simulink model "VehicleDynamicsRing"  (R2020a)
settings: Solver=FixedStepDiscrete  StartTime=0.0  StopTime=10.0  FixedStep=ModelSimTime  RelTol=1e-3  EnableMultiTasking=on
PostLoadFcn:
  | , if any(exist('dsrtsu_mdlpostloadfcn', 'file') ~= 0), dsrtsu_mdlpostloadfcn('Execute', bdroot); end,
InitFcn:
  | , if any(exist('rtifpga_mdlclblib', 'file') ~= 0), rtifpga_mdlclblib('Init', bdroot); end,
undefined symbols (not defined in the file): DRIVE_MODE, VDR
libraries: simulink x4
(part 1 of 2)
settings Model: DSRTSU_INTERNAL_RTI_VER=560  DSRTSU_INTERNAL_RTI_TYPE=rti1401  RTICANMMDATA=struct('GeneralSetupData',struct('modelroot','C:\Users\harjo\Git\MACFormulaGit\MicroAutobox\rings\Vehicle_Dynamics_Ring','generalsettings',struct('filesettings',struct('destfolder',struct('Name','RTICANMM_FILES','Check',1),'buildfolder',struct('Name','.','Check',1),'AbsDestfolder',struct('Name','C:\Users\harjo\Git\MACFormulaGit\MicroAutobox\rings\Vehicle_Dynamics_Ring\RTICANMM_FILES'),'AbsBuildfolder',struct('Name','C:\Users\harjo\Git\MACFormulaGit\MicroAutobox\rings\Vehicle_Dynamics_Ring'))),'options',struct('addpaths',1,'rmpaths',1,'addtrcexclusion',true,'cannavigator',struct('checkmonitoring',0),'show_usrtrc',0,'use_usrtrc',0),'advanced',struct('options',ones(1,100)),'MPSetup',{{}},'RTI',struct('Type','RTI1401','Ver','7.14','Date','02-May-2020'),'modelname','VehicleDynamicsRing','block','VehicleDynamicsRing'))  DSRTSU_INTERNAL_RTIFPGA=160  Creator=Harjot  LastModifiedBy=Harjot
settings DebuggingCC: AlgebraicLoopMsg=error  ArtificialAlgebraicLoopMsg=error  MinStepSizeMsg=error  SFUnexpectedBacktrackingDiag=warning  SFNoUnconditionalDefaultTransitionDiag=warning  SFExecutionAtInitializationDiag=none  ArithmeticOperatorsInVariantConditions=warning
settings HardwareCC: ProdBitPerPointer=32  ProdBitPerSizeT=32  ProdBitPerPtrDiffT=32  ProdLargestAtomicInteger=Integer  ProdEndianess=BigEndian  ProdWordSize=32  ProdHWDeviceType=Custom Processor->Custom  TargetIntDivRoundTo=Zero  TargetEndianess=BigEndian  TargetHWDeviceType=Custom Processor->Custom
settings SFSimCC: SimUseLocalCustomCode=off  MATLABDynamicMemAlloc=off  CustomCodeUndefinedFunction=UseInterfaceOnly
settings RTWCC: Description=dSPACE DS1401 Hardware Platform  SystemTargetFile=rti1401.tlc  MakeCommand=make_rti  TemplateMakefile=rti1401.tmf  RTWUseLocalCustomCode=off
settings CodeAppCC: StateflowObjectComments=on
settings STFCustomTargetCC: UtilityFuncGeneration=Shared location  ParMdlRefBuildCompliant=on  SystemTargetFile=rti1401.tlc
settings GRTTargetCC: TargetLangStandard=C89/C90 (ANSI)  UtilityFuncGeneration=Shared location  CompOptLevelCompliant=off  ConcurrentExecutionCompliant=off  CombineOutputUpdateFcns=off  MatFileLogging=off  CPPClassGenCompliant=off  UseToolchainInfoCompliant=off
settings ConfigComp: CovMetricSettings=dw  CovHtmlReporting=on  CovSaveCumulativeToWorkspaceVar=on  CovSaveSingleToWorkspaceVar=on  CovExternalEMLEnable=off

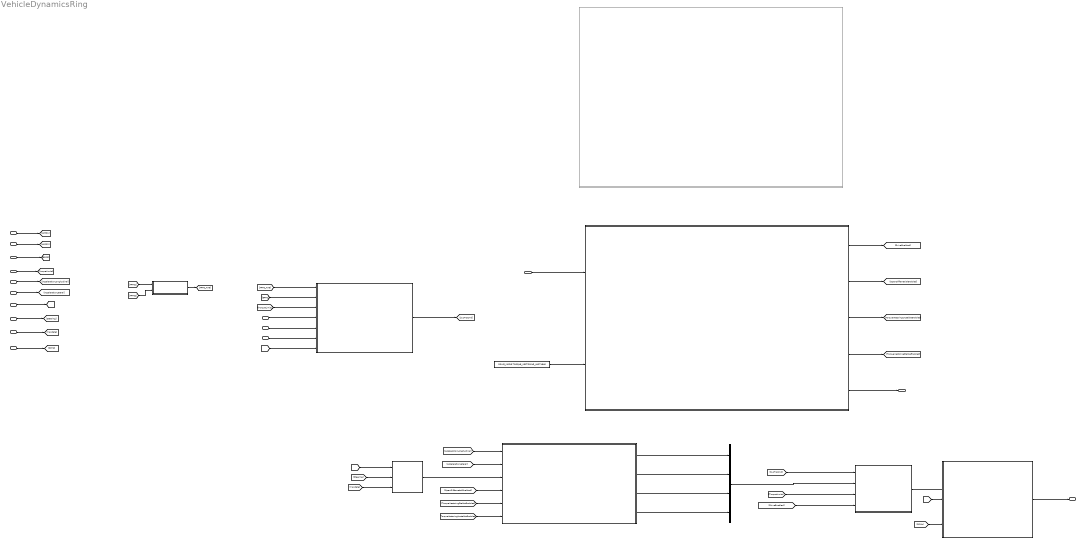
== system VehicleDynamicsRing ==
  VdrModeRequest : Inport  OutDataTypeStr=Enum: MSR_REQUEST
  APPS1 [%]1 : Inport  Port=2  OutDataTypeStr=double
  APPS2 [%]1 : Inport  Port=3  OutDataTypeStr=double
  BPPS : Inport  Port=4  OutDataTypeStr=double
  TorqueLimits : Inport  Port=5  OutDataTypeStr=Bus: TorqueLimits
  AccelerationLongitudinal : Inport  Port=6  OutDataTypeStr=double
  AccelerationLateral : Inport  Port=7  OutDataTypeStr=double
  VehicleSpeed : Inport  Port=8
  SteeringAngle : Inport  Port=9
  YawRate : Inport  Port=10
  ChargeCurrentLimit : Inport  Port=11  OutDataTypeStr=double
  DischargeCurrentLimit : Inport  Port=12  OutDataTypeStr=double
  AccumulatorVoltage : Inport  Port=13
  MotorRPMs : Inport  Port=14  OutDataTypeStr=Bus: MotorRPMs
  APPS Average : Subsystem
  Bus Creator1 : BusCreator  Inputs=4
  Constant1 : Constant  Value=DRIVE_MODE.TORQUE_VECTORING_UNSTABLE
  PedalMapping : ModelReference  ModelNameDialog=PedalMapping.slx  SimulationMode=Normal  ModelReferenceVersion=1.20
  TorqueVectoring : Subsystem
  Traction Control : Subsystem
  VDR Mode Selection : Stateflow chart  TreatAsAtomicUnit=on
  VDR Mode Selection1 : Stateflow chart  Commented=on  TreatAsAtomicUnit=on
  Yaw error subsystem : Subsystem
  torque_distribution_mapping : MATLAB Function  TreatAsAtomicUnit=on
  VdrStatus : Outport  OutDataTypeStr=Enum: RING_STATUS  VectorParamsAs1DForOutWhenUnconnected=off
  TorqueRequests : Outport  Port=2  OutDataTypeStr=Bus: TorqueRequests  VectorParamsAs1DForOutWhenUnconnected=off
  wires:
  VdrModeRequest/1 -> VDR Mode Selection/1(VdrModeRequest)
  AccelerationLongitudinal/1 -> [AccelerationLongitudinal]
  APPS1 [%]1/1 -> [APPS1]
  VehicleSpeed/1 -> [Speed]
  Constant1/1 -> VDR Mode Selection/2(DrivingMode)
  PedalMapping/1 -> [SysTrqCmd]
  APPS Average/1(APPS) -> [APPS_AVG]
  [APPS2] -> APPS Average/2(APPS2)
  APPS2 [%]1/1 -> [APPS2]
  [APPS1] -> APPS Average/1(APPS1)
  BPPS/1 -> [BPPS]
  AccelerationLateral/1 -> [AccelerationLateral]
  DischargeCurrentLimit/1 -> PedalMapping/5
  [APPS_AVG] -> PedalMapping/1
  [BPPS] -> PedalMapping/2
  AccumulatorVoltage/1 -> PedalMapping/6
  [Speed] -> PedalMapping/7
  [TorqueLimits] -> PedalMapping/3
  ChargeCurrentLimit/1 -> PedalMapping/4
  [SysTrqCmd] -> torque_distribution_mapping/1(systemTorque)
  TorqueLimits/1 -> [TorqueLimits]
  [TorqueLimits] -> torque_distribution_mapping/3(torqueLimits)
  Bus Creator1/1 -> torque_distribution_mapping/2(torqueFactors)
  VDR Mode Selection/5(VdrStatus) -> VdrStatus/1  "VDR_Status"
  VDR Mode Selection/4(TorqueVectoringStableEnabled) -> [TorqueVectoringStableEnabled]
  VDR Mode Selection/2(OpenDifferentialEnabled) -> [OpenDiffernetialEnabled]
  [TorqueVectoringStableEnabled] -> TorqueVectoring/5(TorqueVectoringStableEnabled)
  VDR Mode Selection/3(TorqueVectoringUnstableEnabled) -> [TorqueVectoringUnstableEnabled]
  [TorqueVectoringUnstableEnabled] -> TorqueVectoring/6(TorqueVectoringUnstableEnabled)
  Yaw error subsystem/1(Yaw error) -> TorqueVectoring/3(YawError)
  [AccelerationLongitudinal] -> TorqueVectoring/1("AccelerationLongitudinal ")
  [AccelerationLateral] -> TorqueVectoring/2(AccelerationLateral)
  VDR Mode Selection/1(DriveEnabled) -> [DriveEnabled]
  [OpenDiffernetialEnabled] -> TorqueVectoring/4(TorqueVectoringStableEnabled1)
  [Speed] -> Yaw error subsystem/1(Car_speed)
  SteeringAngle/1 -> [Steering]
  [Steering] -> Yaw error subsystem/2(Steering_angle)
  [YawRate] -> Yaw error subsystem/3("Estimated yaw rate ")
  YawRate/1 -> [YawRate]
  [DriveEnabled] -> torque_distribution_mapping/4(driveEnabled)
  TorqueVectoring/1(TorqueScaleRearLeft) -> Bus Creator1/1
  TorqueVectoring/2(TorqueScaleRearRight) -> Bus Creator1/2
  TorqueVectoring/3(TorqueScaleFrontLeft) -> Bus Creator1/3
  TorqueVectoring/4(TorqueScaleFrontRight) -> Bus Creator1/4
  [Speed] -> Traction Control/2(Speed)
  [RPMs] -> Traction Control/3(In3)
  MotorRPMs/1 -> [RPMs]
  Traction Control/1(FinalTorqueRequest) -> TorqueRequests/1
  torque_distribution_mapping/1(torqueRequests) -> Traction Control/1(PreTractionControlTorqueRequest)

== system VehicleDynamicsRing/APPS Average ==
  APPS1 : Inport
  APPS2 : Inport  Port=2
  Add : Sum
  Constant : Constant  Value=2
  Divide : Product  Inputs=*/
  APPS : Outport  VectorParamsAs1DForOutWhenUnconnected=off
  wires:
  Divide/1 -> APPS/1
  APPS2/1 -> Add/2
  APPS1/1 -> Add/1
  Add/1 -> Divide/1
  Constant/1 -> Divide/2

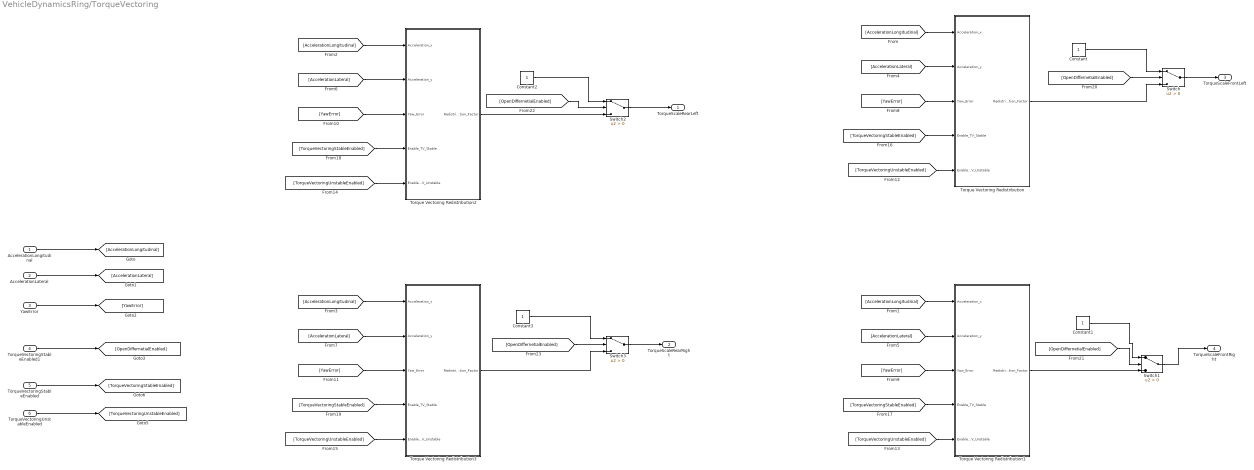
== system VehicleDynamicsRing/TorqueVectoring ==
  "AccelerationLongitudinal " : Inport
  AccelerationLateral : Inport  Port=2
  YawError : Inport  Port=3
  TorqueVectoringStableEnabled1 : Inport  Port=4
  TorqueVectoringStableEnabled : Inport  Port=5
  TorqueVectoringUnstableEnabled : Inport  Port=6
  Constant{,1..3} (4 alike) : Constant
  Switch{,1..3} (4 alike) : Switch  Criteria=u2 > Threshold
  Torque Vectoring Redistribution : Subsystem  AncestorBlock=TorqueVectoringAlgorithmLib/Torque Vectoring Redistribution  mask{wheel_1=Front, wheel_2=Left}
      mask prompts: wheel_1 "Front or Rear Wheel"; wheel_2 "Left or Right Wheel"
      mask init:
      | %Front vs Rear Modifier
      | if(wheel_1 == 1) %Front Wheel
      |     stable_longitudinal_mod = -1;
      | else %Rear Wheel
      |     stable_longitudinal_mod = 1;
      | end
      | 
      | %Left vs Rear Modifier
      | if(wheel_2 == 1) %Left Wheel
      |     unstable_mod = -1;
      |     stable_lateral_mod = -1;
      | else %Right Wheel
      |     unstable_mod = 1;
      |     stable_lateral_mod = 1;
      | end
      mask TypeOptions wheel_1: Front | Rear
      mask TypeOptions wheel_2: Left | Right
      mask DialogControl DescGroupVar Prompt: Torque Vectoring Configurations
      mask DialogControl DescTextVar Prompt: Select the wheel for the torque vectoring configuration.
  Torque Vectoring Redistribution1 : Subsystem  AncestorBlock=TorqueVectoringAlgorithmLib/Torque Vectoring Redistribution  mask{wheel_1=Front, wheel_2=Right}
      mask prompts: wheel_1 "Front or Rear Wheel"; wheel_2 "Left or Right Wheel"
      mask init: same as VehicleDynamicsRing/TorqueVectoring/Torque Vectoring Redistribution
      mask TypeOptions wheel_1: Front | Rear
      mask TypeOptions wheel_2: Left | Right
      mask DialogControl DescGroupVar Prompt: Torque Vectoring Configurations
      mask DialogControl DescTextVar Prompt: Select the wheel for the torque vectoring configuration.
  Torque Vectoring Redistribution2 : Subsystem  AncestorBlock=TorqueVectoringAlgorithmLib/Torque Vectoring Redistribution  mask{wheel_1=Rear, wheel_2=Left}
      mask prompts: wheel_1 "Front or Rear Wheel"; wheel_2 "Left or Right Wheel"
      mask init: same as VehicleDynamicsRing/TorqueVectoring/Torque Vectoring Redistribution
      mask TypeOptions wheel_1: Front | Rear
      mask TypeOptions wheel_2: Left | Right
      mask DialogControl DescGroupVar Prompt: Torque Vectoring Configurations
      mask DialogControl DescTextVar Prompt: Select the wheel for the torque vectoring configuration.
  Torque Vectoring Redistribution3 : Subsystem  AncestorBlock=TorqueVectoringAlgorithmLib/Torque Vectoring Redistribution  mask{wheel_1=Rear, wheel_2=Right}
      mask prompts: wheel_1 "Front or Rear Wheel"; wheel_2 "Left or Right Wheel"
      mask init: same as VehicleDynamicsRing/TorqueVectoring/Torque Vectoring Redistribution
      mask TypeOptions wheel_1: Front | Rear
      mask TypeOptions wheel_2: Left | Right
      mask DialogControl DescGroupVar Prompt: Torque Vectoring Configurations
      mask DialogControl DescTextVar Prompt: Select the wheel for the torque vectoring configuration.
  TorqueScaleRearLeft : Outport  VectorParamsAs1DForOutWhenUnconnected=off
  TorqueScaleRearRight : Outport  Port=2  VectorParamsAs1DForOutWhenUnconnected=off
  TorqueScaleFrontLeft : Outport  Port=3  VectorParamsAs1DForOutWhenUnconnected=off
  TorqueScaleFrontRight : Outport  Port=4  VectorParamsAs1DForOutWhenUnconnected=off
  wires:
  "AccelerationLongitudinal "/1 -> [AccelerationLongitudinal]
  AccelerationLateral/1 -> [AccelerationLateral]
  YawError/1 -> [YawError]
  TorqueVectoringUnstableEnabled/1 -> [TorqueVectoringUnstableEnabled]
  [AccelerationLongitudinal] -> Torque Vectoring Redistribution2/1(Acceleration_x)
  [AccelerationLongitudinal] -> Torque Vectoring Redistribution3/1(Acceleration_x)
  [AccelerationLateral] -> Torque Vectoring Redistribution2/2(Acceleration_y)
  [AccelerationLateral] -> Torque Vectoring Redistribution3/2(Acceleration_y)
  [YawError] -> Torque Vectoring Redistribution2/3(Yaw_Error)
  [YawError] -> Torque Vectoring Redistribution3/3(Yaw_Error)
  TorqueVectoringStableEnabled/1 -> [TorqueVectoringStableEnabled]
  [TorqueVectoringUnstableEnabled] -> Torque Vectoring Redistribution2/5(Enable_TV_Unstable)
  [TorqueVectoringUnstableEnabled] -> Torque Vectoring Redistribution3/5(Enable_TV_Unstable)
  [TorqueVectoringStableEnabled] -> Torque Vectoring Redistribution2/4(Enable_TV_Stable)
  [TorqueVectoringStableEnabled] -> Torque Vectoring Redistribution3/4(Enable_TV_Stable)
  TorqueVectoringStableEnabled1/1 -> [OpenDiffernetialEnabled]
  [TorqueVectoringStableEnabled] -> Torque Vectoring Redistribution/4(Enable_TV_Stable)
  [TorqueVectoringUnstableEnabled] -> Torque Vectoring Redistribution/5(Enable_TV_Unstable)
  [YawError] -> Torque Vectoring Redistribution/3(Yaw_Error)
  [AccelerationLateral] -> Torque Vectoring Redistribution/2(Acceleration_y)
  [AccelerationLongitudinal] -> Torque Vectoring Redistribution/1(Acceleration_x)
  [TorqueVectoringStableEnabled] -> Torque Vectoring Redistribution1/4(Enable_TV_Stable)
  [YawError] -> Torque Vectoring Redistribution1/3(Yaw_Error)
  [AccelerationLongitudinal] -> Torque Vectoring Redistribution1/1(Acceleration_x)
  [TorqueVectoringUnstableEnabled] -> Torque Vectoring Redistribution1/5(Enable_TV_Unstable)
  [AccelerationLateral] -> Torque Vectoring Redistribution1/2(Acceleration_y)
  [OpenDiffernetialEnabled] -> Switch/2
  Switch/1 -> TorqueScaleFrontLeft/1
  [OpenDiffernetialEnabled] -> Switch1/2
  Switch1/1 -> TorqueScaleFrontRight/1
  Constant1/1 -> Switch1/1
  Torque Vectoring Redistribution1/1(Redistribution_Factor) -> Switch1/3
  Torque Vectoring Redistribution/1(Redistribution_Factor) -> Switch/3
  Constant/1 -> Switch/1
  Constant2/1 -> Switch2/1
  [OpenDiffernetialEnabled] -> Switch2/2
  Switch2/1 -> TorqueScaleRearLeft/1
  Torque Vectoring Redistribution2/1(Redistribution_Factor) -> Switch2/3
  Constant3/1 -> Switch3/1
  [OpenDiffernetialEnabled] -> Switch3/2
  Switch3/1 -> TorqueScaleRearRight/1
  Torque Vectoring Redistribution3/1(Redistribution_Factor) -> Switch3/3

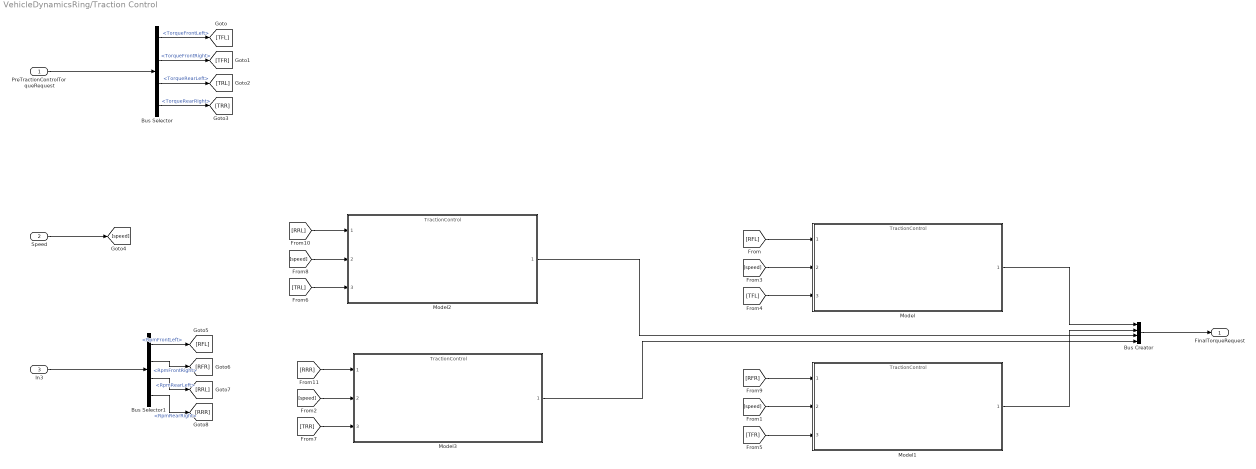
== system VehicleDynamicsRing/Traction Control ==
  PreTractionControlTorqueRequest : Inport
  Speed : Inport  Port=2
  In3 : Inport  Port=3
  Bus Creator : BusCreator  Inputs=4  OutDataTypeStr=Bus: TorqueRequests
  Bus Selector : BusSelector  OutputSignals=TorqueFrontLeft,TorqueFrontRight,TorqueRearLeft,TorqueRearRight
  Bus Selector1 : BusSelector  OutputSignals=RpmFrontLeft,RpmFrontRight,RpmRearLeft,RpmRearRight
  Model{,1..3} (4 alike) : ModelReference  ModelNameDialog=TractionControl.slx  SimulationMode=Normal  ModelReferenceVersion=1.6
  FinalTorqueRequest : Outport  VectorParamsAs1DForOutWhenUnconnected=off
  wires:
  Model3/1 -> Bus Creator/4
  Model2/1 -> Bus Creator/3
  Model1/1 -> Bus Creator/2
  Model/1 -> Bus Creator/1
  Bus Creator/1 -> FinalTorqueRequest/1
  [RFR] -> Model1/1
  [RFL] -> Model/1
  [RRL] -> Model2/1
  [RRR] -> Model3/1
  Bus Selector1/4 -> [RRR]  "<RpmRearRight>"
  Bus Selector1/3 -> [RRL]  "<RpmRearLeft>"
  Bus Selector1/2 -> [RFR]  "<RpmFrontRight>"
  Bus Selector1/1 -> [RFL]  "<RpmFrontLeft>"
  [speed] -> Model1/2
  [speed] -> Model3/2
  [speed] -> Model/2
  [speed] -> Model2/2
  [TRR] -> Model3/3
  [TRL] -> Model2/3
  [TFR] -> Model1/3
  [TFL] -> Model/3
  In3/1 -> Bus Selector1/1
  Speed/1 -> [speed]
  Bus Selector/4 -> [TRR]  "<TorqueRearRight>"
  Bus Selector/3 -> [TRL]  "<TorqueRearLeft>"
  Bus Selector/2 -> [TFR]  "<TorqueFrontRight>"
  Bus Selector/1 -> [TFL]  "<TorqueFrontLeft>"
  PreTractionControlTorqueRequest/1 -> Bus Selector/1

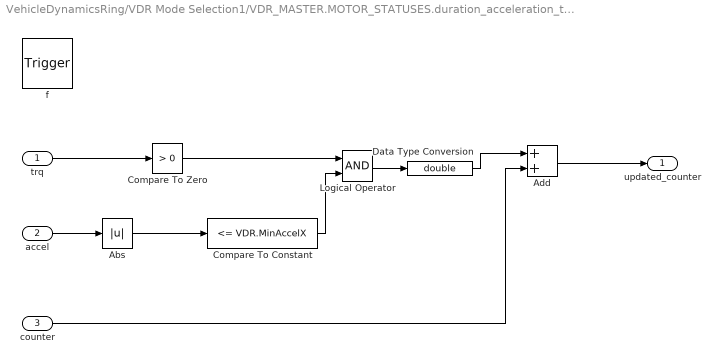
== system VehicleDynamicsRing/VDR Mode Selection1/VDR_MASTER.MOTOR_STATUSES.duration_acceleration_torque_check ==
  trq : Inport  OutDataTypeStr=double  PortDimensions=1
  accel : Inport  Port=2  OutDataTypeStr=double  PortDimensions=1
  counter : Inport  Port=3  OutDataTypeStr=double  PortDimensions=1
  f : TriggerPort  TriggerType=function-call  VariantControl=Variant
      settings: CopyFcn=Stateflow.SLINSF.SimulinkMan.removeBlockPreDeleteFcn  PreDeleteFcn=Stateflow.SLINSF.SimulinkMan.unsafePredeleteFcn
  Abs : Abs
  Add : Sum
  Compare To Constant : simulink/Logic and Bit Operations/Compare To Constant  relop=<=  const=VDR.MinAccelX  OutDataTypeStr=boolean
  Compare To Zero : simulink/Logic and Bit Operations/Compare To Zero  relop=>  OutDataTypeStr=boolean
  Data Type Conversion : DataTypeConversion  OutDataTypeStr=double
  Logical Operator : Logic  AllPortsSameDT=off  OutDataTypeStr=boolean
  updated_counter : Outport  VectorParamsAs1DForOutWhenUnconnected=off
  wires:
  Data Type Conversion/1 -> Add/1
  trq/1 -> Compare To Zero/1
  accel/1 -> Abs/1
  Compare To Zero/1 -> Logical Operator/1
  Compare To Constant/1 -> Logical Operator/2
  Logical Operator/1 -> Data Type Conversion/1
  counter/1 -> Add/2
  Add/1 -> updated_counter/1
  Abs/1 -> Compare To Constant/1

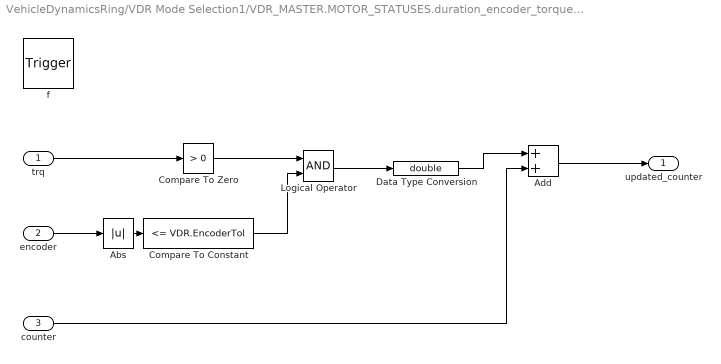
== system VehicleDynamicsRing/VDR Mode Selection1/VDR_MASTER.MOTOR_STATUSES.duration_encoder_torque_check ==
  trq : Inport  OutDataTypeStr=double  PortDimensions=1
  encoder : Inport  Port=2  OutDataTypeStr=double  PortDimensions=1
  counter : Inport  Port=3  OutDataTypeStr=double  PortDimensions=1
  f : TriggerPort  TriggerType=function-call  VariantControl=Variant
      settings: CopyFcn=Stateflow.SLINSF.SimulinkMan.removeBlockPreDeleteFcn  PreDeleteFcn=Stateflow.SLINSF.SimulinkMan.unsafePredeleteFcn
  Abs : Abs
  Add : Sum
  Compare To Constant : simulink/Logic and Bit Operations/Compare To Constant  relop=<=  const=VDR.EncoderTol  OutDataTypeStr=boolean
  Compare To Zero : simulink/Logic and Bit Operations/Compare To Zero  relop=>  OutDataTypeStr=boolean
  Data Type Conversion : DataTypeConversion  OutDataTypeStr=double
  Logical Operator : Logic  AllPortsSameDT=off  OutDataTypeStr=boolean
  updated_counter : Outport  VectorParamsAs1DForOutWhenUnconnected=off
  wires:
  Data Type Conversion/1 -> Add/1
  trq/1 -> Compare To Zero/1
  encoder/1 -> Abs/1
  Compare To Zero/1 -> Logical Operator/1
  Compare To Constant/1 -> Logical Operator/2
  Logical Operator/1 -> Data Type Conversion/1
  counter/1 -> Add/2
  Add/1 -> updated_counter/1
  Abs/1 -> Compare To Constant/1

== system VehicleDynamicsRing/Yaw error subsystem ==
  Car_speed : Inport
  Steering_angle : Inport  Port=2
  "Estimated yaw rate " : Inport  Port=3
  Desired yaw rate calculation : Subsystem
  Subtract : Sum  Inputs=+-
  Yaw rate estimatior : Subsystem  Commented=on
  Yaw error : Outport  VectorParamsAs1DForOutWhenUnconnected=off
  wires:
  Steering_angle/1 -> Desired yaw rate calculation/2(Steering angle)
  Subtract/1 -> Yaw error/1
  "Estimated yaw rate "/1 -> Subtract/2
  Car_speed/1 -> Desired yaw rate calculation/1(Car speed)
  Desired yaw rate calculation/1(Desired yaw rate) -> Subtract/1

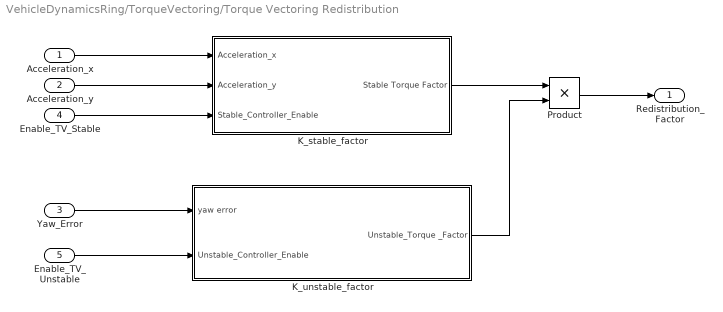
== system VehicleDynamicsRing/TorqueVectoring/Torque Vectoring Redistribution ==
  Acceleration_x : Inport
  Acceleration_y : Inport  Port=2
  Yaw_Error : Inport  Port=3
  Enable_TV_Stable : Inport  Port=4
  Enable_TV_Unstable : Inport  Port=5
  K_stable_factor : Subsystem
  K_unstable_factor : Subsystem
  Product : Product
  Redistribution_Factor : Outport  VectorParamsAs1DForOutWhenUnconnected=off
  wires:
  Enable_TV_Unstable/1 -> K_unstable_factor/2(Unstable_Controller_Enable)
  Enable_TV_Stable/1 -> K_stable_factor/3(Stable_Controller_Enable)
  Product/1 -> Redistribution_Factor/1
  Acceleration_y/1 -> K_stable_factor/2(Acceleration_y)
  Yaw_Error/1 -> K_unstable_factor/1(yaw error)
  Acceleration_x/1 -> K_stable_factor/1(Acceleration_x)
  K_stable_factor/1(Stable Torque Factor) -> Product/1
  K_unstable_factor/1(Unstable_Torque _Factor) -> Product/2

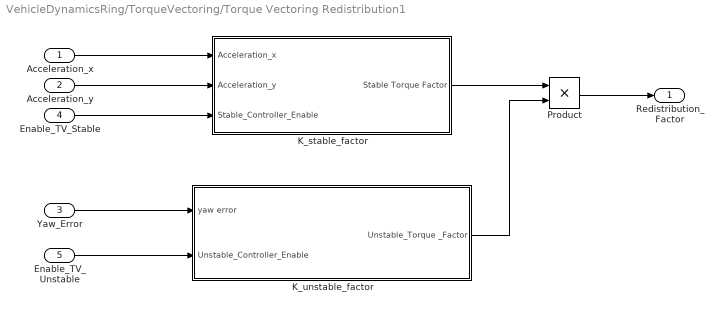
== system VehicleDynamicsRing/TorqueVectoring/Torque Vectoring Redistribution1 ==
  Acceleration_x : Inport
  Acceleration_y : Inport  Port=2
  Yaw_Error : Inport  Port=3
  Enable_TV_Stable : Inport  Port=4
  Enable_TV_Unstable : Inport  Port=5
  K_stable_factor : Subsystem
  K_unstable_factor : Subsystem
  Product : Product
  Redistribution_Factor : Outport  VectorParamsAs1DForOutWhenUnconnected=off
  wires:
  Enable_TV_Unstable/1 -> K_unstable_factor/2(Unstable_Controller_Enable)
  Enable_TV_Stable/1 -> K_stable_factor/3(Stable_Controller_Enable)
  Product/1 -> Redistribution_Factor/1
  Acceleration_y/1 -> K_stable_factor/2(Acceleration_y)
  Yaw_Error/1 -> K_unstable_factor/1(yaw error)
  Acceleration_x/1 -> K_stable_factor/1(Acceleration_x)
  K_stable_factor/1(Stable Torque Factor) -> Product/1
  K_unstable_factor/1(Unstable_Torque _Factor) -> Product/2

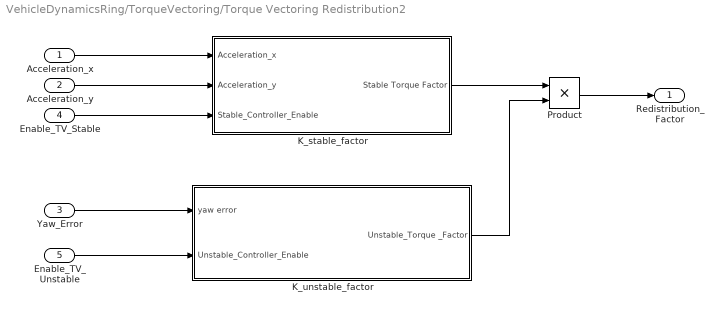
== system VehicleDynamicsRing/TorqueVectoring/Torque Vectoring Redistribution2 ==
  Acceleration_x : Inport
  Acceleration_y : Inport  Port=2
  Yaw_Error : Inport  Port=3
  Enable_TV_Stable : Inport  Port=4
  Enable_TV_Unstable : Inport  Port=5
  K_stable_factor : Subsystem
  K_unstable_factor : Subsystem
  Product : Product
  Redistribution_Factor : Outport  VectorParamsAs1DForOutWhenUnconnected=off
  wires:
  Enable_TV_Unstable/1 -> K_unstable_factor/2(Unstable_Controller_Enable)
  Enable_TV_Stable/1 -> K_stable_factor/3(Stable_Controller_Enable)
  Product/1 -> Redistribution_Factor/1
  Acceleration_y/1 -> K_stable_factor/2(Acceleration_y)
  Yaw_Error/1 -> K_unstable_factor/1(yaw error)
  Acceleration_x/1 -> K_stable_factor/1(Acceleration_x)
  K_stable_factor/1(Stable Torque Factor) -> Product/1
  K_unstable_factor/1(Unstable_Torque _Factor) -> Product/2

== system VehicleDynamicsRing/TorqueVectoring/Torque Vectoring Redistribution3 ==
  Acceleration_x : Inport
  Acceleration_y : Inport  Port=2
  Yaw_Error : Inport  Port=3
  Enable_TV_Stable : Inport  Port=4
  Enable_TV_Unstable : Inport  Port=5
  K_stable_factor : Subsystem
  K_unstable_factor : Subsystem
  Product : Product
  Redistribution_Factor : Outport  VectorParamsAs1DForOutWhenUnconnected=off
  wires:
  Enable_TV_Unstable/1 -> K_unstable_factor/2(Unstable_Controller_Enable)
  Enable_TV_Stable/1 -> K_stable_factor/3(Stable_Controller_Enable)
  Product/1 -> Redistribution_Factor/1
  Acceleration_y/1 -> K_stable_factor/2(Acceleration_y)
  Yaw_Error/1 -> K_unstable_factor/1(yaw error)
  Acceleration_x/1 -> K_stable_factor/1(Acceleration_x)
  K_stable_factor/1(Stable Torque Factor) -> Product/1
  K_unstable_factor/1(Unstable_Torque _Factor) -> Product/2

== system VehicleDynamicsRing/Yaw error subsystem/Desired yaw rate calculation ==
  Car speed : Inport
  Steering angle : Inport  Port=2
  Add : Sum
  "CM to front axel " : Constant  Value=VDR.l_f
  CM to rear axel : Constant  Value=VDR.l_r
  Divide : Product  Inputs=*/
  Product : Product
  Desired yaw rate : Outport  VectorParamsAs1DForOutWhenUnconnected=off
  wires:
  Steering angle/1 -> Product/2
  Add/1 -> Divide/2
  Divide/1 -> Desired yaw rate/1
  Car speed/1 -> Product/1
  Product/1 -> Divide/1
  CM to rear axel/1 -> Add/2
  "CM to front axel "/1 -> Add/1

== system VehicleDynamicsRing/Yaw error subsystem/Yaw rate estimatior ==
  velocity-x : Inport
  steering angle : Inport  Port=2
  Divide : Product  Inputs=*/
  Product : Product
  Trigonometric Function : Trigonometry  Operator=tan
  Wheelbase : Constant  Value=VDR.l
  yaw rate estimate : Outport  VectorParamsAs1DForOutWhenUnconnected=off
  wires:
  steering angle/1 -> Trigonometric Function/1
  velocity-x/1 -> Product/1
  Trigonometric Function/1 -> Product/2
  Product/1 -> Divide/1
  Wheelbase/1 -> Divide/2
  Divide/1 -> yaw rate estimate/1

== system VehicleDynamicsRing/TorqueVectoring/Torque Vectoring Redistribution/K_stable_factor ==
  Acceleration_x : Inport
  Acceleration_y : Inport  Port=2
  Stable_Controller_Enable : Inport  Port=3
  Constant : Constant
  Divide : Product  Inputs=*/
  Switch : Switch  Criteria=u2 > Threshold
  Vehicle Mass : Constant  Value=0.25*VDR.M*VDR.g
  Wheel_Down_Force : Subsystem
  Stable Torque Factor : Outport  VectorParamsAs1DForOutWhenUnconnected=off
  wires:
  Constant/1 -> Switch/3
  Switch/1 -> Stable Torque Factor/1
  Divide/1 -> Switch/1
  Stable_Controller_Enable/1 -> Switch/2
  Vehicle Mass/1 -> Divide/2
  Wheel_Down_Force/1(Stable Weigth Distribution) -> Divide/1
  Acceleration_x/1 -> Wheel_Down_Force/1(Acceleration_x)
  Acceleration_y/1 -> Wheel_Down_Force/2(Acceleration_y)

== system VehicleDynamicsRing/TorqueVectoring/Torque Vectoring Redistribution/K_unstable_factor ==
  yaw error : Inport
  Unstable_Controller_Enable : Inport  Port=2
  Add : Sum
  Constant : Constant
  Constant1 : Constant
  Switch : Switch  Criteria=u2 > Threshold
  Unstable_Controller_Gain : Gain  Gain=VDR.Kp
  Unstable_Modifier : Gain  Gain=unstable_mod
  Unstable_Torque _Factor : Outport  VectorParamsAs1DForOutWhenUnconnected=off
  wires:
  Constant1/1 -> Switch/3
  Unstable_Controller_Enable/1 -> Switch/2
  Switch/1 -> Unstable_Torque _Factor/1
  Add/1 -> Switch/1
  Unstable_Modifier/1 -> Add/1
  yaw error/1 -> Unstable_Controller_Gain/1
  Constant/1 -> Add/2
  Unstable_Controller_Gain/1 -> Unstable_Modifier/1

== system VehicleDynamicsRing/TorqueVectoring/Torque Vectoring Redistribution1/K_stable_factor ==
  Acceleration_x : Inport
  Acceleration_y : Inport  Port=2
  Stable_Controller_Enable : Inport  Port=3
  Constant : Constant
  Divide : Product  Inputs=*/
  Switch : Switch  Criteria=u2 > Threshold
  Vehicle Mass : Constant  Value=0.25*VDR.M*VDR.g
  Wheel_Down_Force : Subsystem
  Stable Torque Factor : Outport  VectorParamsAs1DForOutWhenUnconnected=off
  wires:
  Constant/1 -> Switch/3
  Switch/1 -> Stable Torque Factor/1
  Divide/1 -> Switch/1
  Stable_Controller_Enable/1 -> Switch/2
  Vehicle Mass/1 -> Divide/2
  Wheel_Down_Force/1(Stable Weigth Distribution) -> Divide/1
  Acceleration_x/1 -> Wheel_Down_Force/1(Acceleration_x)
  Acceleration_y/1 -> Wheel_Down_Force/2(Acceleration_y)

== system VehicleDynamicsRing/TorqueVectoring/Torque Vectoring Redistribution1/K_unstable_factor ==
  yaw error : Inport
  Unstable_Controller_Enable : Inport  Port=2
  Add : Sum
  Constant : Constant
  Constant1 : Constant
  Switch : Switch  Criteria=u2 > Threshold
  Unstable_Controller_Gain : Gain  Gain=VDR.Kp
  Unstable_Modifier : Gain  Gain=unstable_mod
  Unstable_Torque _Factor : Outport  VectorParamsAs1DForOutWhenUnconnected=off
  wires:
  Constant1/1 -> Switch/3
  Unstable_Controller_Enable/1 -> Switch/2
  Switch/1 -> Unstable_Torque _Factor/1
  Add/1 -> Switch/1
  Unstable_Modifier/1 -> Add/1
  yaw error/1 -> Unstable_Controller_Gain/1
  Constant/1 -> Add/2
  Unstable_Controller_Gain/1 -> Unstable_Modifier/1

== system VehicleDynamicsRing/TorqueVectoring/Torque Vectoring Redistribution2/K_stable_factor ==
  Acceleration_x : Inport
  Acceleration_y : Inport  Port=2
  Stable_Controller_Enable : Inport  Port=3
  Constant : Constant
  Divide : Product  Inputs=*/
  Switch : Switch  Criteria=u2 > Threshold
  Vehicle Mass : Constant  Value=0.25*VDR.M*VDR.g
  Wheel_Down_Force : Subsystem
  Stable Torque Factor : Outport  VectorParamsAs1DForOutWhenUnconnected=off
  wires:
  Constant/1 -> Switch/3
  Switch/1 -> Stable Torque Factor/1
  Divide/1 -> Switch/1
  Stable_Controller_Enable/1 -> Switch/2
  Vehicle Mass/1 -> Divide/2
  Wheel_Down_Force/1(Stable Weigth Distribution) -> Divide/1
  Acceleration_x/1 -> Wheel_Down_Force/1(Acceleration_x)
  Acceleration_y/1 -> Wheel_Down_Force/2(Acceleration_y)

== system VehicleDynamicsRing/TorqueVectoring/Torque Vectoring Redistribution2/K_unstable_factor ==
  yaw error : Inport
  Unstable_Controller_Enable : Inport  Port=2
  Add : Sum
  Constant : Constant
  Constant1 : Constant
  Switch : Switch  Criteria=u2 > Threshold
  Unstable_Controller_Gain : Gain  Gain=VDR.Kp
  Unstable_Modifier : Gain  Gain=unstable_mod
  Unstable_Torque _Factor : Outport  VectorParamsAs1DForOutWhenUnconnected=off
  wires:
  Constant1/1 -> Switch/3
  Unstable_Controller_Enable/1 -> Switch/2
  Switch/1 -> Unstable_Torque _Factor/1
  Add/1 -> Switch/1
  Unstable_Modifier/1 -> Add/1
  yaw error/1 -> Unstable_Controller_Gain/1
  Constant/1 -> Add/2
  Unstable_Controller_Gain/1 -> Unstable_Modifier/1

== system VehicleDynamicsRing/TorqueVectoring/Torque Vectoring Redistribution3/K_stable_factor ==
  Acceleration_x : Inport
  Acceleration_y : Inport  Port=2
  Stable_Controller_Enable : Inport  Port=3
  Constant : Constant
  Divide : Product  Inputs=*/
  Switch : Switch  Criteria=u2 > Threshold
  Vehicle Mass : Constant  Value=0.25*VDR.M*VDR.g
  Wheel_Down_Force : Subsystem
  Stable Torque Factor : Outport  VectorParamsAs1DForOutWhenUnconnected=off
  wires:
  Constant/1 -> Switch/3
  Switch/1 -> Stable Torque Factor/1
  Divide/1 -> Switch/1
  Stable_Controller_Enable/1 -> Switch/2
  Vehicle Mass/1 -> Divide/2
  Wheel_Down_Force/1(Stable Weigth Distribution) -> Divide/1
  Acceleration_x/1 -> Wheel_Down_Force/1(Acceleration_x)
  Acceleration_y/1 -> Wheel_Down_Force/2(Acceleration_y)

== system VehicleDynamicsRing/TorqueVectoring/Torque Vectoring Redistribution3/K_unstable_factor ==
  yaw error : Inport
  Unstable_Controller_Enable : Inport  Port=2
  Add : Sum
  Constant : Constant
  Constant1 : Constant
  Switch : Switch  Criteria=u2 > Threshold
  Unstable_Controller_Gain : Gain  Gain=VDR.Kp
  Unstable_Modifier : Gain  Gain=unstable_mod
  Unstable_Torque _Factor : Outport  VectorParamsAs1DForOutWhenUnconnected=off
  wires:
  Constant1/1 -> Switch/3
  Unstable_Controller_Enable/1 -> Switch/2
  Switch/1 -> Unstable_Torque _Factor/1
  Add/1 -> Switch/1
  Unstable_Modifier/1 -> Add/1
  yaw error/1 -> Unstable_Controller_Gain/1
  Constant/1 -> Add/2
  Unstable_Controller_Gain/1 -> Unstable_Modifier/1

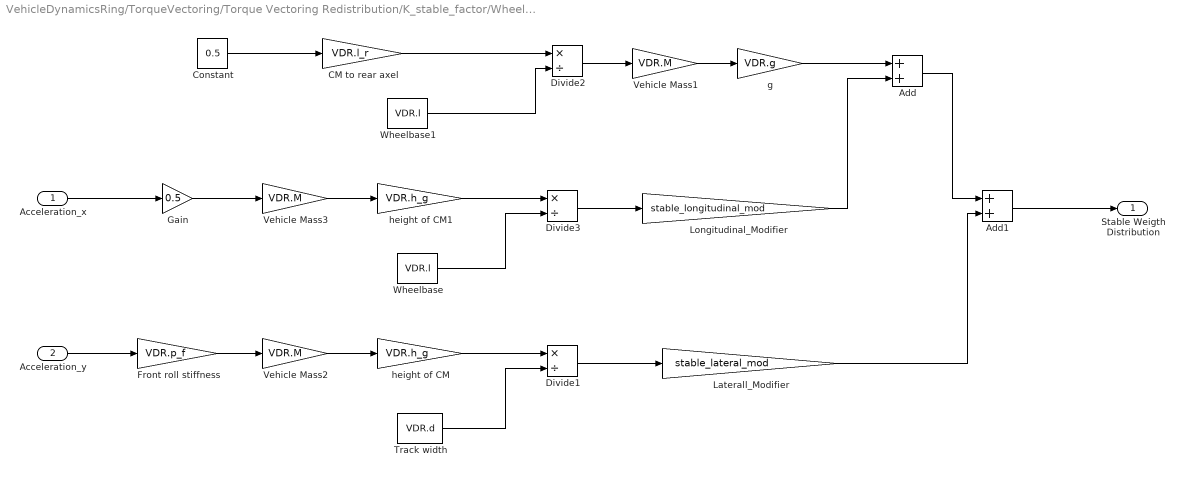
== system VehicleDynamicsRing/TorqueVectoring/Torque Vectoring Redistribution/K_stable_factor/Wheel_Down_Force ==
  Acceleration_x : Inport
  Acceleration_y : Inport  Port=2
  Add : Sum
  Add1 : Sum
  CM to rear axel : Gain  Gain=VDR.l_r
  Constant : Constant  Value=0.5
  Divide1 : Product  Inputs=*/
  Divide2 : Product  Inputs=*/
  Divide3 : Product  Inputs=*/
  Front roll stiffness : Gain  Gain=VDR.p_f
  Gain : Gain  Gain=0.5
  Laterall_Modifier : Gain  Gain=stable_lateral_mod
  Longitudinal_Modifier : Gain  Gain=stable_longitudinal_mod
  Track width : Constant  Value=VDR.d
  Vehicle Mass1 : Gain  Gain=VDR.M
  Vehicle Mass2 : Gain  Gain=VDR.M
  Vehicle Mass3 : Gain  Gain=VDR.M
  Wheelbase : Constant  Value=VDR.l
  Wheelbase1 : Constant  Value=VDR.l
  g : Gain  Gain=VDR.g
  height of CM : Gain  Gain=VDR.h_g
  height of CM1 : Gain  Gain=VDR.h_g
  Stable Weigth Distribution : Outport  VectorParamsAs1DForOutWhenUnconnected=off
  wires:
  Gain/1 -> Vehicle Mass3/1
  Laterall_Modifier/1 -> Add1/2
  Add/1 -> Add1/1
  Longitudinal_Modifier/1 -> Add/2
  g/1 -> Add/1
  Track width/1 -> Divide1/2
  Wheelbase/1 -> Divide3/2
  Divide1/1 -> Laterall_Modifier/1
  Divide3/1 -> Longitudinal_Modifier/1
  Wheelbase1/1 -> Divide2/2
  Divide2/1 -> Vehicle Mass1/1
  Acceleration_y/1 -> Front roll stiffness/1
  Constant/1 -> CM to rear axel/1
  CM to rear axel/1 -> Divide2/1
  Acceleration_x/1 -> Gain/1
  Front roll stiffness/1 -> Vehicle Mass2/1
  Vehicle Mass1/1 -> g/1
  Vehicle Mass2/1 -> height of CM/1
  height of CM/1 -> Divide1/1
  Vehicle Mass3/1 -> height of CM1/1
  height of CM1/1 -> Divide3/1
  Add1/1 -> Stable Weigth Distribution/1

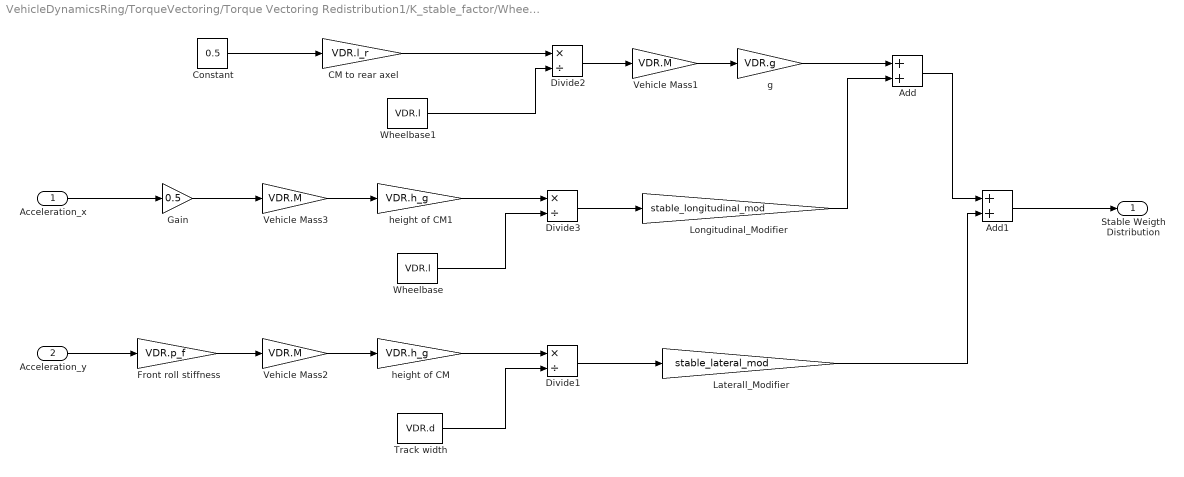
== system VehicleDynamicsRing/TorqueVectoring/Torque Vectoring Redistribution1/K_stable_factor/Wheel_Down_Force ==
  Acceleration_x : Inport
  Acceleration_y : Inport  Port=2
  Add : Sum
  Add1 : Sum
  CM to rear axel : Gain  Gain=VDR.l_r
  Constant : Constant  Value=0.5
  Divide1 : Product  Inputs=*/
  Divide2 : Product  Inputs=*/
  Divide3 : Product  Inputs=*/
  Front roll stiffness : Gain  Gain=VDR.p_f
  Gain : Gain  Gain=0.5
  Laterall_Modifier : Gain  Gain=stable_lateral_mod
  Longitudinal_Modifier : Gain  Gain=stable_longitudinal_mod
  Track width : Constant  Value=VDR.d
  Vehicle Mass1 : Gain  Gain=VDR.M
  Vehicle Mass2 : Gain  Gain=VDR.M
  Vehicle Mass3 : Gain  Gain=VDR.M
  Wheelbase : Constant  Value=VDR.l
  Wheelbase1 : Constant  Value=VDR.l
  g : Gain  Gain=VDR.g
  height of CM : Gain  Gain=VDR.h_g
  height of CM1 : Gain  Gain=VDR.h_g
  Stable Weigth Distribution : Outport  VectorParamsAs1DForOutWhenUnconnected=off
  wires:
  Gain/1 -> Vehicle Mass3/1
  Laterall_Modifier/1 -> Add1/2
  Add/1 -> Add1/1
  Longitudinal_Modifier/1 -> Add/2
  g/1 -> Add/1
  Track width/1 -> Divide1/2
  Wheelbase/1 -> Divide3/2
  Divide1/1 -> Laterall_Modifier/1
  Divide3/1 -> Longitudinal_Modifier/1
  Wheelbase1/1 -> Divide2/2
  Divide2/1 -> Vehicle Mass1/1
  Acceleration_y/1 -> Front roll stiffness/1
  Constant/1 -> CM to rear axel/1
  CM to rear axel/1 -> Divide2/1
  Acceleration_x/1 -> Gain/1
  Front roll stiffness/1 -> Vehicle Mass2/1
  Vehicle Mass1/1 -> g/1
  Vehicle Mass2/1 -> height of CM/1
  height of CM/1 -> Divide1/1
  Vehicle Mass3/1 -> height of CM1/1
  height of CM1/1 -> Divide3/1
  Add1/1 -> Stable Weigth Distribution/1

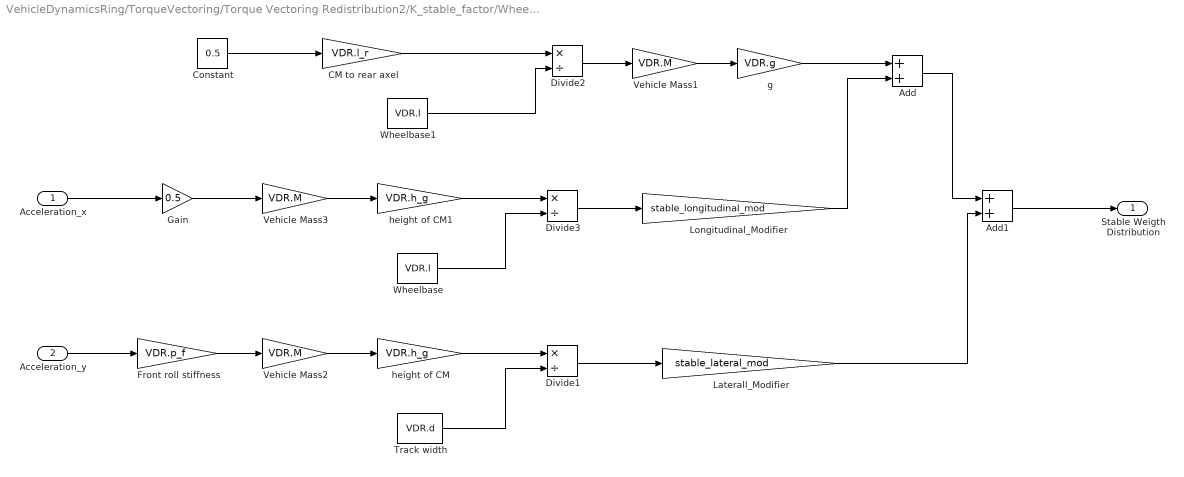
== system VehicleDynamicsRing/TorqueVectoring/Torque Vectoring Redistribution2/K_stable_factor/Wheel_Down_Force ==
  Acceleration_x : Inport
  Acceleration_y : Inport  Port=2
  Add : Sum
  Add1 : Sum
  CM to rear axel : Gain  Gain=VDR.l_r
  Constant : Constant  Value=0.5
  Divide1 : Product  Inputs=*/
  Divide2 : Product  Inputs=*/
  Divide3 : Product  Inputs=*/
  Front roll stiffness : Gain  Gain=VDR.p_f
  Gain : Gain  Gain=0.5
  Laterall_Modifier : Gain  Gain=stable_lateral_mod
  Longitudinal_Modifier : Gain  Gain=stable_longitudinal_mod
  Track width : Constant  Value=VDR.d
  Vehicle Mass1 : Gain  Gain=VDR.M
  Vehicle Mass2 : Gain  Gain=VDR.M
  Vehicle Mass3 : Gain  Gain=VDR.M
  Wheelbase : Constant  Value=VDR.l
  Wheelbase1 : Constant  Value=VDR.l
  g : Gain  Gain=VDR.g
  height of CM : Gain  Gain=VDR.h_g
  height of CM1 : Gain  Gain=VDR.h_g
  Stable Weigth Distribution : Outport  VectorParamsAs1DForOutWhenUnconnected=off
  wires:
  Gain/1 -> Vehicle Mass3/1
  Laterall_Modifier/1 -> Add1/2
  Add/1 -> Add1/1
  Longitudinal_Modifier/1 -> Add/2
  g/1 -> Add/1
  Track width/1 -> Divide1/2
  Wheelbase/1 -> Divide3/2
  Divide1/1 -> Laterall_Modifier/1
  Divide3/1 -> Longitudinal_Modifier/1
  Wheelbase1/1 -> Divide2/2
  Divide2/1 -> Vehicle Mass1/1
  Acceleration_y/1 -> Front roll stiffness/1
  Constant/1 -> CM to rear axel/1
  CM to rear axel/1 -> Divide2/1
  Acceleration_x/1 -> Gain/1
  Front roll stiffness/1 -> Vehicle Mass2/1
  Vehicle Mass1/1 -> g/1
  Vehicle Mass2/1 -> height of CM/1
  height of CM/1 -> Divide1/1
  Vehicle Mass3/1 -> height of CM1/1
  height of CM1/1 -> Divide3/1
  Add1/1 -> Stable Weigth Distribution/1

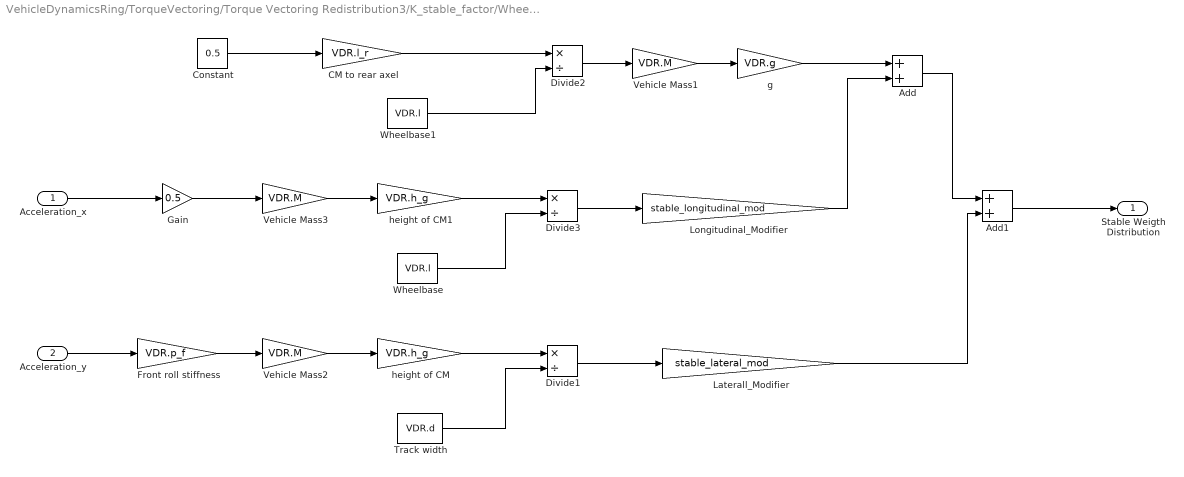
== system VehicleDynamicsRing/TorqueVectoring/Torque Vectoring Redistribution3/K_stable_factor/Wheel_Down_Force ==
  Acceleration_x : Inport
  Acceleration_y : Inport  Port=2
  Add : Sum
  Add1 : Sum
  CM to rear axel : Gain  Gain=VDR.l_r
  Constant : Constant  Value=0.5
  Divide1 : Product  Inputs=*/
  Divide2 : Product  Inputs=*/
  Divide3 : Product  Inputs=*/
  Front roll stiffness : Gain  Gain=VDR.p_f
  Gain : Gain  Gain=0.5
  Laterall_Modifier : Gain  Gain=stable_lateral_mod
  Longitudinal_Modifier : Gain  Gain=stable_longitudinal_mod
  Track width : Constant  Value=VDR.d
  Vehicle Mass1 : Gain  Gain=VDR.M
  Vehicle Mass2 : Gain  Gain=VDR.M
  Vehicle Mass3 : Gain  Gain=VDR.M
  Wheelbase : Constant  Value=VDR.l
  Wheelbase1 : Constant  Value=VDR.l
  g : Gain  Gain=VDR.g
  height of CM : Gain  Gain=VDR.h_g
  height of CM1 : Gain  Gain=VDR.h_g
  Stable Weigth Distribution : Outport  VectorParamsAs1DForOutWhenUnconnected=off
  wires:
  Gain/1 -> Vehicle Mass3/1
  Laterall_Modifier/1 -> Add1/2
  Add/1 -> Add1/1
  Longitudinal_Modifier/1 -> Add/2
  g/1 -> Add/1
  Track width/1 -> Divide1/2
  Wheelbase/1 -> Divide3/2
  Divide1/1 -> Laterall_Modifier/1
  Divide3/1 -> Longitudinal_Modifier/1
  Wheelbase1/1 -> Divide2/2
  Divide2/1 -> Vehicle Mass1/1
  Acceleration_y/1 -> Front roll stiffness/1
  Constant/1 -> CM to rear axel/1
  CM to rear axel/1 -> Divide2/1
  Acceleration_x/1 -> Gain/1
  Front roll stiffness/1 -> Vehicle Mass2/1
  Vehicle Mass1/1 -> g/1
  Vehicle Mass2/1 -> height of CM/1
  height of CM/1 -> Divide1/1
  Vehicle Mass3/1 -> height of CM1/1
  height of CM1/1 -> Divide3/1
  Add1/1 -> Stable Weigth Distribution/1
